simulink model "Q_3_BilinearHPF"  (R2020b)
settings: Solver=VariableStepDiscrete  StartTime=0.0  StopTime=0.05  MaxStep=0.00000021008403361344539  RelTol=1e-3
values from neighbouring files (symbols this model uses):
  a0 = 1.0    [data_dict.sldd]
  a1 = 0.1584    [data_dict.sldd]
  b0 = 0.5792    [data_dict.sldd]
  b1 = -0.5792    [data_dict.sldd]
undefined symbols (not defined in the file or in its folder): rc
settings Model: DataDictionary=data_dict.sldd  Creator=Shree  LastModifiedBy=Shree

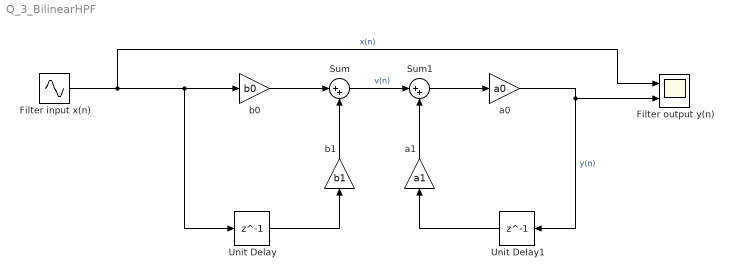
== system Q_3_BilinearHPF ==
  Filter input x(n) : Sin  Amplitude=2  Frequency=rc  SampleTime=0
  Filter output y(n) : Scope  NumInputPorts=2
  Sum : Sum  Inputs=|++
  Sum1 : Sum  Inputs=|++
  Unit Delay : Delay  DelayLength=1  InitialCondition=0
  Unit Delay1 : Delay  DelayLength=1  InitialCondition=0
  a0 : Gain  Gain=a0
  a1 : Gain  Gain=a1
  b0 : Gain  Gain=b0
  b1 : Gain  Gain=b1
  wires:
  Sum/1 -> Sum1/1  "v(n)"
  Unit Delay/1 -> b1/1
  Unit Delay1/1 -> a1/1
  Sum1/1 -> a0/1
  b0/1 -> Sum/1
  b1/1 -> Sum/2
  a0/1 -> Filter output y(n)/2, Unit Delay1/1  "y(n)"
  a1/1 -> Sum1/2
  Filter input x(n)/1 -> Filter output y(n)/1, Unit Delay/1, b0/1  "x(n)"
